simulink model "Analysis_model_MOD"  (R2025b)
settings: Solver=ode2  StartTime=0.0  StopTime=Tf  FixedStep=Tstep  RelTol=1e-3
values from neighbouring files (symbols this model uses):
  Km = 12.4132 / 12.7177    (= 0.976056991437)    [Stabilization_MOD.m]
  Kp = (2*W_cl*Zeta_cl*Time_const - 1)/Km    [Stabilization_MOD.m]
  Sim_disturbance_freq = pi    (= 3.14159265359)    [Stabilization_MOD.m]
  Sim_saturation_neg = -20    [Stabilization_MOD.m]
  Sim_saturation_pos = 20    [Stabilization_MOD.m]
  Time_const = 1 / 12.7177    (= 0.078630569993)    [Stabilization_MOD.m]
  Tsample = 0.005    [Stabilization_MOD.m]
undefined symbols (not defined in the file or in its folder): DiscIntNeverNeededParam
settings Model: Creator=GILBERT  LastModifiedBy=GILBERT

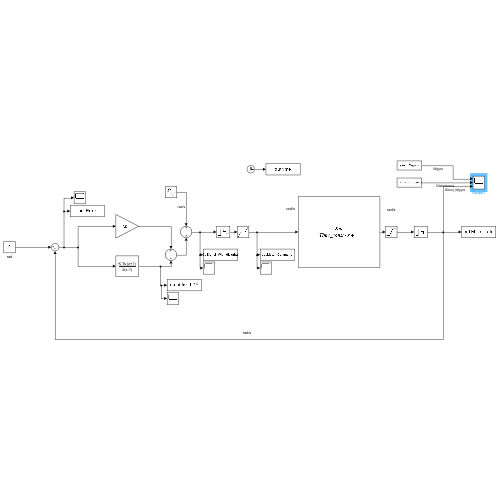
[thumbnail: Simulink's stored preview of the top-level diagram]
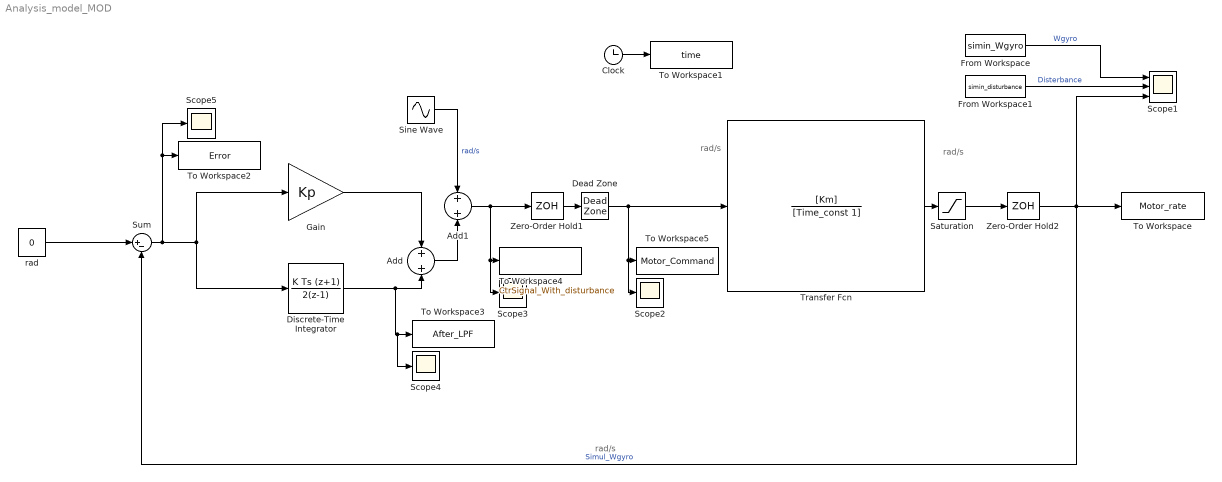
== system Analysis_model_MOD ==
  note: rad/s
  note: rad/s
  note: rad/s
  Add : Sum
  Add1 : Sum
  Clock : Clock
  Dead Zone : DeadZone  LowerValue=Sim_deadZone_start  UpperValue=Sim_deadZone_final
  Discrete-Time Integrator : DiscreteIntegrator  IntegratorMethod=Integration: Trapezoidal  gainval=Ki  SampleTime=Tsample  ICPrevOutput=DiscIntNeverNeededParam  ICPrevScaledInput=DiscIntNeverNeededParam
  From Workspace : FromWorkspace  VariableName=simin_Wgyro  SampleTime=Tsample
  From Workspace1 : FromWorkspace  VariableName=simin_disturbance  SampleTime=Tsample
  Gain : Gain  Gain=Kp
  Saturation : Saturate  UpperLimit=Sim_saturation_pos  LowerLimit=Sim_saturation_neg
  Scope1 : Scope  NumInputPorts=3
      settings: ActiveDisplayYMinimum=-29.503801096346479  ActiveDisplayYMaximum=3.5903635948564006
  Scope{2..5} (4 alike) : Scope
      Scope2 settings: ActiveDisplayYMinimum=-1.1644474527973081  ActiveDisplayYMaximum=1.0939827146871717
      Scope3 settings: ActiveDisplayYMinimum=-2.1275872286509654  ActiveDisplayYMaximum=1.543670912095062  DataLoggingVariableName=ScopeData2
      Scope4 settings: ActiveDisplayYMinimum=-9.5219105166274414  ActiveDisplayYMaximum=9.5219105166274414  DataLoggingVariableName=ScopeData3
      Scope5 settings: ActiveDisplayYMinimum=-1.1644474527973081  ActiveDisplayYMaximum=1.0939827146871717  DataLoggingVariableName=ScopeData4
  Sine Wave : Sin  Amplitude=4.5  Frequency=Sim_disturbance_freq  SampleTime=Tsample
  Sum : Sum  Inputs=|+-
  To Workspace : ToWorkspace  VariableName=Motor_rate  SampleTime=-1
  To Workspace1 : ToWorkspace  VariableName=time  SampleTime=-1
  To Workspace2 : ToWorkspace  VariableName=Error  SampleTime=-1
  To Workspace3 : ToWorkspace  VariableName=After_LPF  SampleTime=-1
  To Workspace4 : ToWorkspace  VariableName=CtrSignal_With_disturbance  SampleTime=-1
  To Workspace5 : ToWorkspace  VariableName=Motor_Command  SampleTime=-1
  Transfer Fcn : TransferFcn  Numerator=[Km]  Denominator=[Time_const 1]
  Zero-Order Hold1 : ZeroOrderHold  SampleTime=Tsample
  Zero-Order Hold2 : ZeroOrderHold  SampleTime=Tsample
  rad : Constant  Value=0
  wires:
  Gain/1 -> Add/1
  Add/1 -> Add1/2
  Sine Wave/1 -> Add1/1  "rad/s"
  Sum/1 -> To Workspace2/1, Scope5/1, Discrete-Time Integrator/1, Gain/1
  rad/1 -> Sum/1
  Add1/1 -> Scope3/1, To Workspace4/1, Zero-Order Hold1/1
  Discrete-Time Integrator/1 -> Scope4/1, To Workspace3/1, Add/2
  Zero-Order Hold1/1 -> Dead Zone/1
  Dead Zone/1 -> Scope2/1, To Workspace5/1, Transfer Fcn/1
  Saturation/1 -> Zero-Order Hold2/1
  Zero-Order Hold2/1 -> To Workspace/1, Scope1/3, Sum/2  "Simul_Wgyro"
  Clock/1 -> To Workspace1/1
  Transfer Fcn/1 -> Saturation/1
  From Workspace1/1 -> Scope1/2  "Disterbance"
  From Workspace/1 -> Scope1/1  "Wgyro"
